simulink model "Exp4_1"  (R2024a)
settings: Solver=ode1  StartTime=0.0  StopTime=10.0  FixedStep=1e-4  RelTol=1e-3
model workspace (MAT data in the model file):
  tau = Simulink.Parameter
  tau.Complexity = 'real'
  tau.Dimensions = [0 0]
  tau.DataType = 'auto'
settings Model: LastModifiedBy=Rodrigo

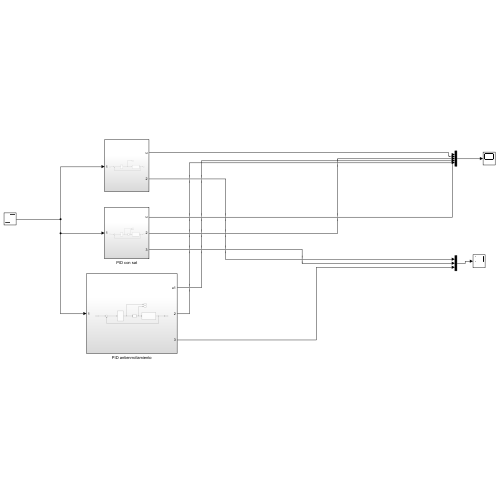
[thumbnail: Simulink's stored preview of the top-level diagram]
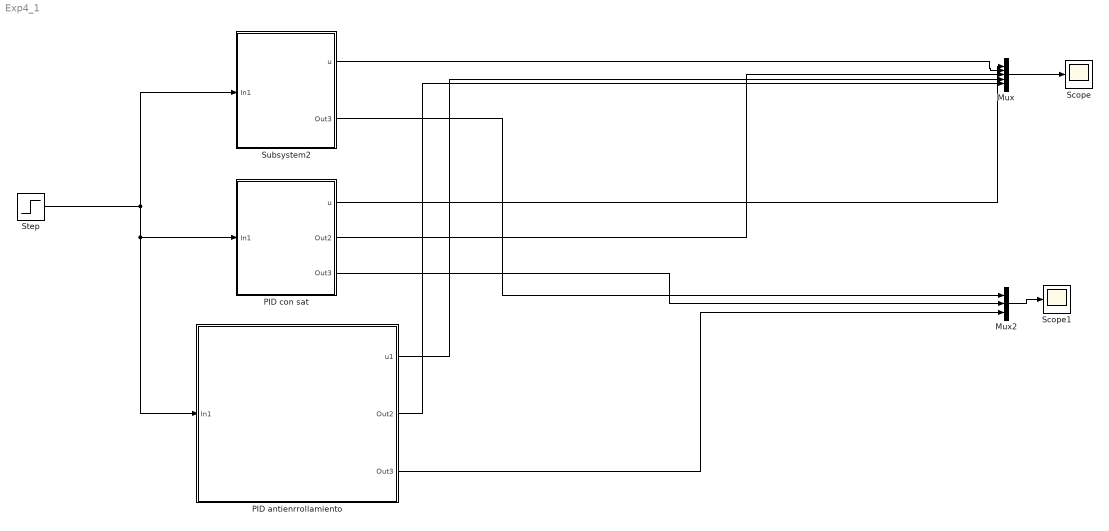
== system Exp4_1 ==
  Mux : Mux  Inputs=5
  Mux2 : Mux  Inputs=3
  PID antienrrollamiento : Subsystem
  PID con sat : Subsystem
  Scope : Scope
  Scope1 : Scope
  Step : Step  After=.8  SampleTime=0
  Subsystem2 : Subsystem
  wires:
  Mux/1 -> Scope/1
  PID antienrrollamiento/3(Out3) -> Mux2/3
  PID con sat/3(Out3) -> Mux2/2
  Subsystem2/2(Out3) -> Mux2/1
  Subsystem2/1(u) -> Mux/2
  PID con sat/1(u) -> Mux/1
  PID con sat/2(Out2) -> Mux/3
  PID antienrrollamiento/1(u1) -> Mux/4
  PID antienrrollamiento/2(Out2) -> Mux/5
  Mux2/1 -> Scope1/1
  Step/1 -> PID antienrrollamiento/1(In1), PID con sat/1(In1), Subsystem2/1(In1)

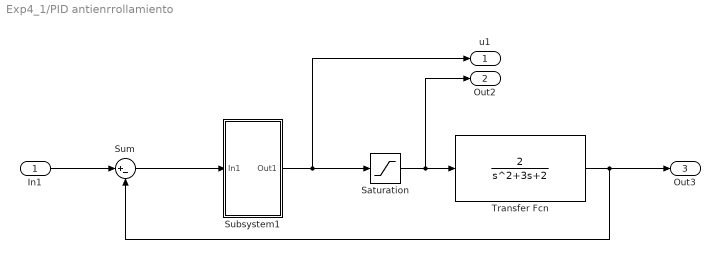
== system Exp4_1/PID antienrrollamiento ==
  In1 : Inport
  Saturation : Saturate  UpperLimit=1  LowerLimit=-1
  Subsystem1 : Subsystem  mask{KP=5.67, KD=.93, KI=8, tau=1/9.09, Umax=1, Umin=-1}
  Sum : Sum  Inputs=|+-
  Transfer Fcn : TransferFcn  Numerator=[2]  Denominator=[1 3 2]
  u1 : Outport
  Out2 : Outport  Port=2
  Out3 : Outport  Port=3
  wires:
  Transfer Fcn/1 -> Out3/1, Sum/2
  Subsystem1/1(Out1) -> u1/1, Saturation/1
  Saturation/1 -> Out2/1, Transfer Fcn/1
  Sum/1 -> Subsystem1/1(In1)
  In1/1 -> Sum/1

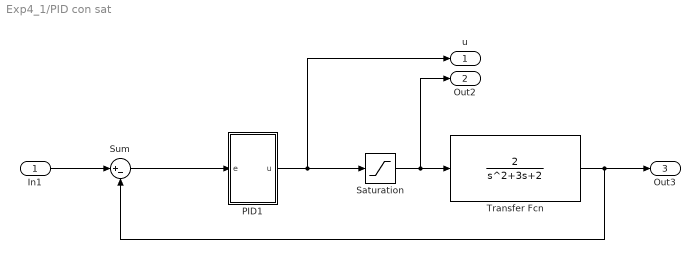
== system Exp4_1/PID con sat ==
  In1 : Inport
  PID1 : Subsystem  mask{KP=5.67, KI=8, KD=0.93, tau=1/9.09}
  Saturation : Saturate  UpperLimit=1  LowerLimit=-1
  Sum : Sum  Inputs=|+-
  Transfer Fcn : TransferFcn  Numerator=[2]  Denominator=[1 3 2]
  u : Outport
  Out2 : Outport  Port=2
  Out3 : Outport  Port=3
  wires:
  Saturation/1 -> Out2/1, Transfer Fcn/1
  PID1/1(u) -> u/1, Saturation/1
  In1/1 -> Sum/1
  Sum/1 -> PID1/1(e)
  Transfer Fcn/1 -> Out3/1, Sum/2

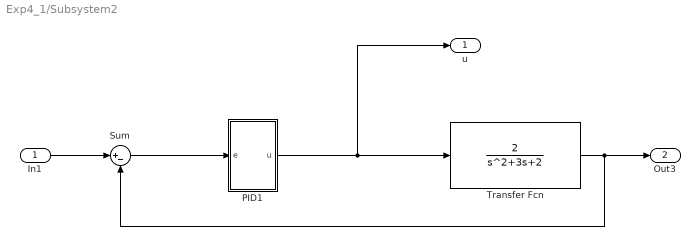
== system Exp4_1/Subsystem2 ==
  In1 : Inport
  PID1 : Subsystem  mask{KP=5.67, KI=8, KD=0.93, tau=1/9.09}
  Sum : Sum  Inputs=|+-
  Transfer Fcn : TransferFcn  Numerator=[2]  Denominator=[1 3 2]
  u : Outport
  Out3 : Outport  Port=2
  wires:
  PID1/1(u) -> u/1, Transfer Fcn/1
  In1/1 -> Sum/1
  Sum/1 -> PID1/1(e)
  Transfer Fcn/1 -> Out3/1, Sum/2

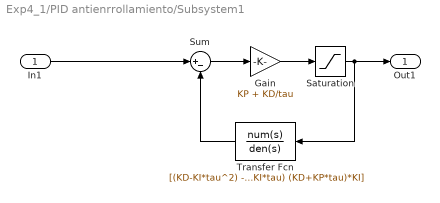
== system Exp4_1/PID antienrrollamiento/Subsystem1 ==
  In1 : Inport
  Gain : Gain  Gain=KP + KD/tau
  Saturation : Saturate  UpperLimit=Umax  LowerLimit=Umin
  Sum : Sum  Inputs=|+-
  Transfer Fcn : TransferFcn  Numerator=[(KD-KI*tau^2) -(tau*KI)]  Denominator=[(KD+KP*tau)^2 (KD+KP*tau)*(KP+KI*tau) (KD+KP*tau)*KI]
  Out1 : Outport
  wires:
  In1/1 -> Sum/1
  Saturation/1 -> Out1/1, Transfer Fcn/1
  Gain/1 -> Saturation/1
  Sum/1 -> Gain/1
  Transfer Fcn/1 -> Sum/2

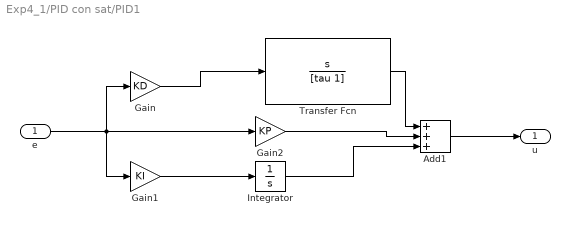
== system Exp4_1/PID con sat/PID1 ==
  e : Inport
  Add1 : Sum  Inputs=+++
  Gain : Gain  Gain=KD
  Gain1 : Gain  Gain=KI
  Gain2 : Gain  Gain=KP
  Integrator : Integrator
  Transfer Fcn : TransferFcn  Numerator=[1 0]  Denominator=[tau 1]
  u : Outport
  wires:
  Gain/1 -> Transfer Fcn/1
  e/1 -> Gain/1, Gain1/1, Gain2/1
  Add1/1 -> u/1
  Integrator/1 -> Add1/3
  Gain2/1 -> Add1/2
  Transfer Fcn/1 -> Add1/1
  Gain1/1 -> Integrator/1

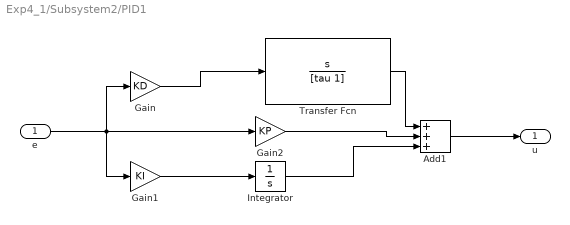
== system Exp4_1/Subsystem2/PID1 ==
  e : Inport
  Add1 : Sum  Inputs=+++
  Gain : Gain  Gain=KD
  Gain1 : Gain  Gain=KI
  Gain2 : Gain  Gain=KP
  Integrator : Integrator
  Transfer Fcn : TransferFcn  Numerator=[1 0]  Denominator=[tau 1]
  u : Outport
  wires:
  Gain/1 -> Transfer Fcn/1
  e/1 -> Gain/1, Gain1/1, Gain2/1
  Add1/1 -> u/1
  Integrator/1 -> Add1/3
  Gain2/1 -> Add1/2
  Transfer Fcn/1 -> Add1/1
  Gain1/1 -> Integrator/1
